simulink model "continuouscontrol"  (R2013b)
settings: Solver=ode45  StartTime=0.0  StopTime=10.0  RelTol=1e-3
undefined symbols (not defined in the file): a, b, c, K
settings Model: Creator=tvincent  LastModifiedBy=tvincent

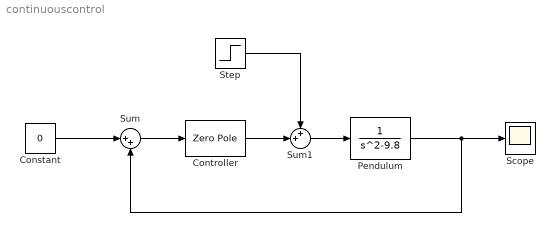
== system continuouscontrol ==
  Constant : Constant  Value=0
  Controller : ZeroPole  Zeros=[-a]  Poles=[-b c]  Gain=K
  Pendulum : TransferFcn  Denominator=[1 0 -9.8]
  Scope : Scope
  Step : Step  SampleTime=0
  Sum : Sum  Inputs=|++
  Sum1 : Sum  Inputs=++|
  wires:
  Pendulum/1 -> Sum/2, Scope/1
  Sum/1 -> Controller/1
  Constant/1 -> Sum/1
  Sum1/1 -> Pendulum/1
  Controller/1 -> Sum1/2
  Step/1 -> Sum1/1
